simulink model "lab9_test"  (R2024a)
settings: Solver=VariableStepAuto  StartTime=0.0  StopTime=1000  RelTol=1e-3
values from neighbouring files (symbols this model uses):
  m = m + 1    (= 2)    [lab5.m]
undefined symbols (not defined in the file or in its folder): n
settings Model: Creator=QQshnik  LastModifiedBy=QQshnik
settings SolverCC: AlgebraicLoopSolver=TrustRegion
settings DataIOCC: SaveOutput=off  SaveTime=off
settings DebuggingCC: UnconnectedInputMsg=warning  UnconnectedOutputMsg=warning  UnconnectedLineMsg=warning  ArithmeticOperatorsInVariantConditions=warning
settings ModelReferenceCC: EnableRefExpFcnMdlSchedulingChecks=on
settings SFSimCC: SimUseLocalCustomCode=off  CustomCodeUndefinedFunction=UseInterfaceOnly
settings RTWCC: RTWUseLocalCustomCode=off  GPUComputeCapability=3.5
settings CodeAppCC: StateflowObjectComments=on

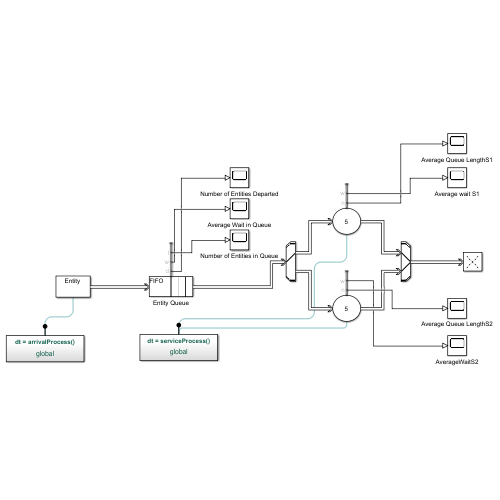
[thumbnail: Simulink's stored preview of the top-level diagram]
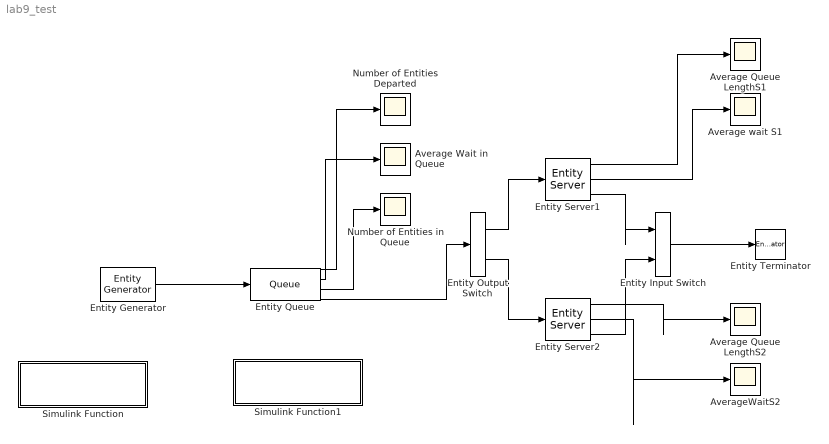
== system lab9_test ==
  Average Queue LengthS1 : Scope
  Average Queue LengthS2 : Scope
  Average Wait in Queue : Scope
  Average wait S1 : Scope
  AverageWaitS2 : Scope
  Entity Input Switch : EntityInputSwitch  InputPortMessageModes=m,m  OutputPortMessageModes=m
  Entity Output Switch : EntityOutputSwitch  InputPortMessageModes=m  OutputPortMessageModes=m,m  SwitchingCriterion=Equiprobable  SwitchAttributeName=Attribute1  InitialPortSelection=2
  Entity Generator : EntityGenerator  OutputPortMessageModes=m  TimeSource=MATLAB action  IntergenerationTimeAction=dt = arrivalProcess();  EntityType=Structured  EntityTypeName=Entity
  Entity Queue : Queue  InputPortMessageModes=m  OutputPortMessageModes=n,n,n,m  Capacity=1  NumberEntitiesDeparted=on  AverageWait=on  AverageQueueLength=on
      settings: OutputPortMap=o0,o2,o3,o5
  Entity Server1 : EntityServer  InputPortMessageModes=m  OutputPortMessageModes=n,n,m  ServiceTimeSource=MATLAB action  ServiceTimeAction=dt = serviceProcess();  NumberEntitiesInBlock=on  AverageWait=on
      settings: OutputPortMap=o1,o4,o9
  Entity Server2 : EntityServer  InputPortMessageModes=m  OutputPortMessageModes=n,n,m  ServiceTimeSource=MATLAB action  ServiceTimeAction=dt = serviceProcess();  NumberEntitiesInBlock=on  AverageWait=on
      settings: OutputPortMap=o1,o4,o9
  Entity Terminator : EntityTerminator  InputPortMessageModes=m
  Number of Entities Departed : Scope
  Number of Entities in Queue : Scope
  Simulink Function : Subsystem  TreatAsAtomicUnit=on
  Simulink Function1 : Subsystem  TreatAsAtomicUnit=on
  wires:
  Entity Queue/2 -> Average Wait in Queue/1
  Entity Queue/1 -> Number of Entities Departed/1
  Entity Output Switch/1 -> Entity Server1/1
  Entity Output Switch/2 -> Entity Server2/1
  Entity Server1/3 -> Entity Input Switch/1
  Entity Server2/3 -> Entity Input Switch/2
  Entity Input Switch/1 -> Entity Terminator/1
  Entity Server1/2 -> Average wait S1/1
  Entity Server2/2 -> AverageWaitS2/1
  Entity Server2/1 -> Average Queue LengthS2/1
  Entity Server1/1 -> Average Queue LengthS1/1
  Entity Queue/3 -> Number of Entities in Queue/1
  Entity Generator/1 -> Entity Queue/1
  Entity Queue/4 -> Entity Output Switch/1

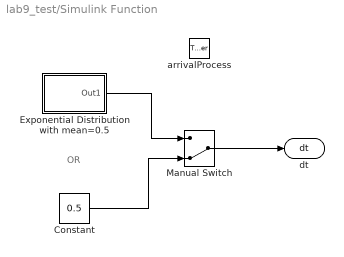
== system lab9_test/Simulink Function ==
  note: OR
  arrivalProcess : TriggerPort  TriggerType=function-call  IsSimulinkFunction=on  FunctionName=arrivalProcess  VariantControl=Variant
  Constant : Constant  Value=0.5
  Exponential Distribution with mean=0.5 : Subsystem
  Manual Switch : ManualSwitch  CurrentSetting=0
  dt : ArgOut  DisableCoverage=on  ArgumentName=dt
  wires:
  Manual Switch/1 -> dt/1
  Exponential Distribution with mean=0.5/1(Out1) -> Manual Switch/1
  Constant/1 -> Manual Switch/2

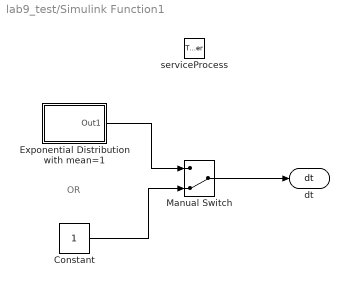
== system lab9_test/Simulink Function1 ==
  note: OR
  serviceProcess : TriggerPort  TriggerType=function-call  IsSimulinkFunction=on  FunctionName=serviceProcess  VariantControl=Variant
  Constant : Constant
  Exponential Distribution with mean=1 : Subsystem
  Manual Switch : ManualSwitch  CurrentSetting=0
  dt : ArgOut  DisableCoverage=on  ArgumentName=dt
  wires:
  Manual Switch/1 -> dt/1
  Constant/1 -> Manual Switch/2
  Exponential Distribution with mean=1/1(Out1) -> Manual Switch/1

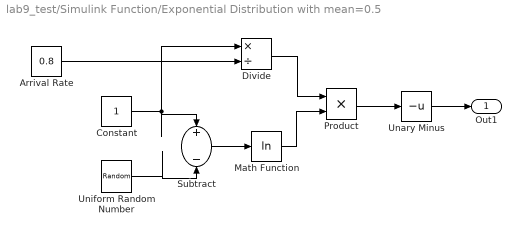
== system lab9_test/Simulink Function/Exponential Distribution with mean=0.5 ==
  Arrival Rate : Constant  Value=0.8
  Constant : Constant
  Divide : Product  Inputs=*/
  Math Function : Math  Operator=log
  Product : Product
  Subtract : Sum  Inputs=+-
  Unary Minus : UnaryMinus
  Uniform Random Number : UniformRandomNumber  Minimum=0  Seed=12345
  Out1 : Outport
  wires:
  Unary Minus/1 -> Out1/1
  Arrival Rate/1 -> Divide/2
  Divide/1 -> Product/1
  Subtract/1 -> Math Function/1
  Math Function/1 -> Product/2
  Product/1 -> Unary Minus/1
  Uniform Random Number/1 -> Subtract/2
  Constant/1 -> Divide/1, Subtract/1

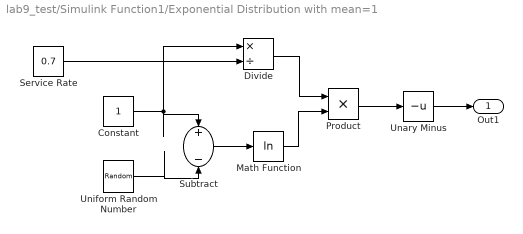
== system lab9_test/Simulink Function1/Exponential Distribution with mean=1 ==
  Constant : Constant
  Divide : Product  Inputs=*/
  Math Function : Math  Operator=log
  Product : Product
  Service Rate : Constant  Value=0.7
  Subtract : Sum  Inputs=+-
  Unary Minus : UnaryMinus
  Uniform Random Number : UniformRandomNumber  Minimum=0  Seed=98765
  Out1 : Outport
  wires:
  Unary Minus/1 -> Out1/1
  Service Rate/1 -> Divide/2
  Divide/1 -> Product/1
  Subtract/1 -> Math Function/1
  Math Function/1 -> Product/2
  Product/1 -> Unary Minus/1
  Uniform Random Number/1 -> Subtract/2
  Constant/1 -> Divide/1, Subtract/1
